simulink model "ASM1_Influentmodel_calibration"  (Simulink 7.6)
settings: Solver=ode45  StartTime=0.0  StopTime=730  RelTol=1e-6
values from neighbouring files (symbols this model uses):
  aHpercent = 75    [ASM1_Influent_init.m]    (also in ASM1_Influent_init_MC_IBU.m; ASM1_Influent_init_MC_T.m; ASM1_Influent_init_MC_TSS.m; ASM1_Influent_init_dry.m)
  CODpart_gperPEperd = 115.08    [ASM1_Influent_init.m]    (also in ASM1_Influent_init_MC_IBU.m; ASM1_Influent_init_MC_T.m = 80; ASM1_Influent_init_MC_TSS.m = RandomMatrix1(a,1); ASM1_Influent_init_dry.m)
  CODpart_HH_max = 20*CODpart_gperPEperd*PE    (= 184128)    [ASM1_Influent_init.m]    (also in ASM1_Influent_init_MC_IBU.m = 36825.6; ASM1_Influent_init_MC_T.m = 25600; ASM1_Influent_init_MC_TSS.m = 20*CODpart_gperPEperd*PE; ASM1_Influent_init_dry.m = 36825.6)
  CODpart_HH_min = 0.1    [ASM1_Influent_init.m]    (also in ASM1_Influent_init_MC_IBU.m; ASM1_Influent_init_MC_T.m; ASM1_Influent_init_MC_TSS.m; ASM1_Influent_init_dry.m)
  CODpart_HH_ns = 35000    [ASM1_Influent_init.m]    (also in ASM1_Influent_init_MC_IBU.m; ASM1_Influent_init_MC_T.m; ASM1_Influent_init_MC_TSS.m; ASM1_Influent_init_dry.m)
  CODpart_HH_nv = factor1*CODpart_gperPEperd*PE    (= 18412.8)    [ASM1_Influent_init.m]    (also in ASM1_Influent_init_MC_IBU.m = 3682.56; ASM1_Influent_init_MC_T.m = 2560; ASM1_Influent_init_MC_TSS.m = factor1*CODpart_gperPEperd*PE; ASM1_Influent_init_dry.m = 3682.56)
  CODpart_HH_st = 1/24    (= 0.0416666666667)    [ASM1_Influent_init.m]    (also in ASM1_Influent_init_MC_IBU.m; ASM1_Influent_init_MC_T.m; ASM1_Influent_init_MC_TSS.m; ASM1_Influent_init_dry.m)
  CODpart_Ind_kgperd = 2301.80    (= 2301.8)    [ASM1_Influent_init.m]    (also in ASM1_Influent_init_MC_IBU.m = 0; ASM1_Influent_init_MC_T.m = 0; ASM1_Influent_init_MC_TSS.m = 0; ASM1_Influent_init_dry.m)
  CODpart_Ind_max = 20*CODpart_Ind_kgperd    (= 46036)    [ASM1_Influent_init.m]    (also in ASM1_Influent_init_MC_IBU.m = 20; ASM1_Influent_init_MC_T.m = 20; ASM1_Influent_init_MC_TSS.m = 20; ASM1_Influent_init_dry.m)
  CODpart_Ind_min = 0.1    [ASM1_Influent_init.m]    (also in ASM1_Influent_init_MC_IBU.m; ASM1_Influent_init_MC_T.m; ASM1_Influent_init_MC_TSS.m; ASM1_Influent_init_dry.m)
  CODpart_Ind_ns = 21000    [ASM1_Influent_init.m]    (also in ASM1_Influent_init_MC_IBU.m; ASM1_Influent_init_MC_T.m; ASM1_Influent_init_MC_TSS.m; ASM1_Influent_init_dry.m)
  CODpart_Ind_nv = factor2*CODpart_Ind_kgperd    (= 4603.6)    [ASM1_Influent_init.m]    (also in ASM1_Influent_init_MC_IBU.m = 0; ASM1_Influent_init_MC_T.m = 0; ASM1_Influent_init_MC_TSS.m = 0; ASM1_Influent_init_dry.m)
  CODpart_Ind_st = 1/24    (= 0.0416666666667)    [ASM1_Influent_init.m]    (also in ASM1_Influent_init_MC_IBU.m; ASM1_Influent_init_MC_T.m; ASM1_Influent_init_MC_TSS.m; ASM1_Influent_init_dry.m)
  CODsol_gperPEperd = 19.31    [ASM1_Influent_init.m]    (also in ASM1_Influent_init_MC_IBU.m; ASM1_Influent_init_MC_T.m; ASM1_Influent_init_MC_TSS.m; ASM1_Influent_init_dry.m)
  CODsol_HH_max = 20*CODsol_gperPEperd*PE    (= 30896)    [ASM1_Influent_init.m]    (also in ASM1_Influent_init_MC_IBU.m = 6179.2; ASM1_Influent_init_MC_T.m = 6179.2; ASM1_Influent_init_MC_TSS.m = 6179.2; ASM1_Influent_init_dry.m = 6179.2)
  CODsol_HH_min = 0.1    [ASM1_Influent_init.m]    (also in ASM1_Influent_init_MC_IBU.m; ASM1_Influent_init_MC_T.m; ASM1_Influent_init_MC_TSS.m; ASM1_Influent_init_dry.m)
  CODsol_HH_ns = 25000    [ASM1_Influent_init.m]    (also in ASM1_Influent_init_MC_IBU.m; ASM1_Influent_init_MC_T.m; ASM1_Influent_init_MC_TSS.m; ASM1_Influent_init_dry.m)
  CODsol_HH_nv = factor1*2*CODsol_gperPEperd*PE    (= 6179.2)    [ASM1_Influent_init.m]    (also in ASM1_Influent_init_MC_IBU.m = 1235.84; ASM1_Influent_init_MC_T.m = 1235.84; ASM1_Influent_init_MC_TSS.m = 1235.84; ASM1_Influent_init_dry.m = 1235.84)
  CODsol_HH_st = 1/24    (= 0.0416666666667)    [ASM1_Influent_init.m]    (also in ASM1_Influent_init_MC_IBU.m; ASM1_Influent_init_MC_T.m; ASM1_Influent_init_MC_TSS.m; ASM1_Influent_init_dry.m)
  CODsol_Ind_kgperd = 386.24    [ASM1_Influent_init.m]    (also in ASM1_Influent_init_MC_IBU.m = 0; ASM1_Influent_init_MC_T.m = 0; ASM1_Influent_init_MC_TSS.m = 0; ASM1_Influent_init_dry.m)
  CODsol_Ind_max = 20*CODsol_Ind_kgperd    (= 7724.8)    [ASM1_Influent_init.m]    (also in ASM1_Influent_init_MC_IBU.m = 20; ASM1_Influent_init_MC_T.m = 20; ASM1_Influent_init_MC_TSS.m = 20; ASM1_Influent_init_dry.m)
  CODsol_Ind_min = 0.1    [ASM1_Influent_init.m]    (also in ASM1_Influent_init_MC_IBU.m; ASM1_Influent_init_MC_T.m; ASM1_Influent_init_MC_TSS.m; ASM1_Influent_init_dry.m)
  CODsol_Ind_ns = 11000    [ASM1_Influent_init.m]    (also in ASM1_Influent_init_MC_IBU.m; ASM1_Influent_init_MC_T.m; ASM1_Influent_init_MC_TSS.m; ASM1_Influent_init_dry.m)
  CODsol_Ind_nv = factor2*CODsol_Ind_kgperd    (= 772.48)    [ASM1_Influent_init.m]    (also in ASM1_Influent_init_MC_IBU.m = 0; ASM1_Influent_init_MC_T.m = 0; ASM1_Influent_init_MC_TSS.m = 0; ASM1_Influent_init_dry.m)
  CODsol_Ind_st = 1/24    (= 0.0416666666667)    [ASM1_Influent_init.m]    (also in ASM1_Influent_init_MC_IBU.m; ASM1_Influent_init_MC_T.m; ASM1_Influent_init_MC_TSS.m; ASM1_Influent_init_dry.m)
  FFfraction = 0.25    [ASM1_Influent_init.m]    (also in ASM1_Influent_init_MC_IBU.m; ASM1_Influent_init_MC_T.m = 0.4; ASM1_Influent_init_MC_TSS.m = RandomMatrix1(a,2); ASM1_Influent_init_dry.m)
  HHnoiseswitch = 1    [ASM1_Influent_init.m]    (also in ASM1_Influent_init_MC_IBU.m; ASM1_Influent_init_MC_T.m; ASM1_Influent_init_MC_TSS.m; ASM1_Influent_init_dry.m)
  HHpolnoiseswitch = 1    [ASM1_Influent_init.m]    (also in ASM1_Influent_init_MC_IBU.m; ASM1_Influent_init_MC_T.m; ASM1_Influent_init_MC_TSS.m; ASM1_Influent_init_dry.m)
  HHpopswitch = 100    [ASM1_Influent_init.m]    (also in ASM1_Influent_init_MC_IBU.m; ASM1_Influent_init_MC_T.m; ASM1_Influent_init_MC_TSS.m; ASM1_Influent_init_dry.m)
  Indnoiseswitch = 1    [ASM1_Influent_init.m]    (also in ASM1_Influent_init_MC_IBU.m; ASM1_Influent_init_MC_T.m; ASM1_Influent_init_MC_TSS.m; ASM1_Influent_init_dry.m)
  Indpolnoiseswitch = 1    [ASM1_Influent_init.m]    (also in ASM1_Influent_init_MC_IBU.m; ASM1_Influent_init_MC_T.m; ASM1_Influent_init_MC_TSS.m; ASM1_Influent_init_dry.m)
  Indpopswitch = 100    [ASM1_Influent_init.m]    (also in ASM1_Influent_init_MC_IBU.m; ASM1_Influent_init_MC_T.m = 0; ASM1_Influent_init_MC_TSS.m = 0; ASM1_Influent_init_dry.m)
  InfAmp = 1200    [ASM1_Influent_init.m]    (also in ASM1_Influent_init_MC_IBU.m; ASM1_Influent_init_MC_T.m; ASM1_Influent_init_MC_TSS.m; ASM1_Influent_init_dry.m)
  InfBias = 7100    [ASM1_Influent_init.m]    (also in ASM1_Influent_init_MC_IBU.m; ASM1_Influent_init_MC_T.m; ASM1_Influent_init_MC_TSS.m; ASM1_Influent_init_dry.m)
  Infcst = 7100    [ASM1_Influent_init.m]    (also in ASM1_Influent_init_MC_IBU.m; ASM1_Influent_init_MC_T.m; ASM1_Influent_init_MC_TSS.m; ASM1_Influent_init_dry.m)
  InfFreq = 2*pi/364    (= 0.0172614980966)    [ASM1_Influent_init.m]    (also in ASM1_Influent_init_MC_IBU.m; ASM1_Influent_init_MC_T.m; ASM1_Influent_init_MC_TSS.m; ASM1_Influent_init_dry.m)
  InfPhase = -pi*15/24    (= -1.96349540849)    [ASM1_Influent_init.m]    (also in ASM1_Influent_init_MC_IBU.m; ASM1_Influent_init_MC_T.m; ASM1_Influent_init_MC_TSS.m; ASM1_Influent_init_dry.m)
  PE = 80    [ASM1_Influent_init.m]    (also in ASM1_Influent_init_MC_IBU.m = 16; ASM1_Influent_init_MC_T.m = 16; ASM1_Influent_init_MC_TSS.m = 16; ASM1_Influent_init_dry.m = 16)
  polnoiseswitch = 1    [ASM1_Influent_init.m]    (also in ASM1_Influent_init_MC_IBU.m; ASM1_Influent_init_MC_T.m; ASM1_Influent_init_MC_TSS.m; ASM1_Influent_init_dry.m)
  Q_HH_ns = 3857    [ASM1_Influent_init.m]    (also in ASM1_Influent_init_MC_IBU.m; ASM1_Influent_init_MC_T.m; ASM1_Influent_init_MC_TSS.m; ASM1_Influent_init_dry.m)
  Q_HH_nv = 4000    [ASM1_Influent_init.m]    (also in ASM1_Influent_init_MC_IBU.m; ASM1_Influent_init_MC_T.m; ASM1_Influent_init_MC_TSS.m; ASM1_Influent_init_dry.m)
  Q_HH_st = 1/24    (= 0.0416666666667)    [ASM1_Influent_init.m]    (also in ASM1_Influent_init_MC_IBU.m; ASM1_Influent_init_MC_T.m; ASM1_Influent_init_MC_TSS.m; ASM1_Influent_init_dry.m)
  Q_Ind_ns = 2000    [ASM1_Influent_init.m]    (also in ASM1_Influent_init_MC_IBU.m; ASM1_Influent_init_MC_T.m; ASM1_Influent_init_MC_TSS.m; ASM1_Influent_init_dry.m)
  Q_Ind_nv = 15000    [ASM1_Influent_init.m]    (also in ASM1_Influent_init_MC_IBU.m; ASM1_Influent_init_MC_T.m; ASM1_Influent_init_MC_TSS.m; ASM1_Influent_init_dry.m)
  Q_Ind_st = 1/24    (= 0.0416666666667)    [ASM1_Influent_init.m]    (also in ASM1_Influent_init_MC_IBU.m; ASM1_Influent_init_MC_T.m; ASM1_Influent_init_MC_TSS.m; ASM1_Influent_init_dry.m)
  Q_SCI_ns = 1000    [ASM1_Influent_init.m]    (also in ASM1_Influent_init_MC_IBU.m; ASM1_Influent_init_MC_T.m; ASM1_Influent_init_MC_TSS.m; ASM1_Influent_init_dry.m)
  Q_SCI_nv = 0.1*InfBias    (= 710)    [ASM1_Influent_init.m]    (also in ASM1_Influent_init_MC_IBU.m; ASM1_Influent_init_MC_T.m; ASM1_Influent_init_MC_TSS.m; ASM1_Influent_init_dry.m)
  Q_SCI_st = 1    [ASM1_Influent_init.m]    (also in ASM1_Influent_init_MC_IBU.m; ASM1_Influent_init_MC_T.m; ASM1_Influent_init_MC_TSS.m; ASM1_Influent_init_dry.m)
  QHHsatmax = QperPE*50    (= 7500)    [ASM1_Influent_init.m]    (also in ASM1_Influent_init_MC_IBU.m; ASM1_Influent_init_MC_T.m; ASM1_Influent_init_MC_TSS.m; ASM1_Influent_init_dry.m)
  QHHsatmin = 0.001    [ASM1_Influent_init.m]    (also in ASM1_Influent_init_MC_IBU.m; ASM1_Influent_init_MC_T.m; ASM1_Influent_init_MC_TSS.m; ASM1_Influent_init_dry.m)
  QInd_weekday = 2500    [ASM1_Influent_init.m]    (also in ASM1_Influent_init_MC_IBU.m; ASM1_Influent_init_MC_T.m; ASM1_Influent_init_MC_TSS.m; ASM1_Influent_init_dry.m)
  QIndsatmax = QInd_weekday*10    (= 25000)    [ASM1_Influent_init.m]    (also in ASM1_Influent_init_MC_IBU.m; ASM1_Influent_init_MC_T.m; ASM1_Influent_init_MC_TSS.m; ASM1_Influent_init_dry.m)
  QIndsatmin = 0.001    [ASM1_Influent_init.m]    (also in ASM1_Influent_init_MC_IBU.m; ASM1_Influent_init_MC_T.m; ASM1_Influent_init_MC_TSS.m; ASM1_Influent_init_dry.m)
  Qpermm = 1500    [ASM1_Influent_init.m]    (also in ASM1_Influent_init_MC_IBU.m; ASM1_Influent_init_MC_T.m; ASM1_Influent_init_MC_TSS.m; ASM1_Influent_init_dry.m)
  QperPE = 150    [ASM1_Influent_init.m]    (also in ASM1_Influent_init_MC_IBU.m; ASM1_Influent_init_MC_T.m; ASM1_Influent_init_MC_TSS.m; ASM1_Influent_init_dry.m)
  QSCIsatmax = 2*(InfBias+InfAmp)    (= 16600)    [ASM1_Influent_init.m]    (also in ASM1_Influent_init_MC_IBU.m; ASM1_Influent_init_MC_T.m; ASM1_Influent_init_MC_TSS.m; ASM1_Influent_init_dry.m)
  QSCIsatmin = 0.0    (= 0)    [ASM1_Influent_init.m]    (also in ASM1_Influent_init_MC_IBU.m; ASM1_Influent_init_MC_T.m; ASM1_Influent_init_MC_TSS.m; ASM1_Influent_init_dry.m)
  rainpopswitch = 100    [ASM1_Influent_init.m]    (also in ASM1_Influent_init_MC_IBU.m = 0; ASM1_Influent_init_MC_T.m = 0; ASM1_Influent_init_MC_TSS.m = 0; ASM1_Influent_init_dry.m = 0)
  SCInoiseswitch = 0    [ASM1_Influent_init.m]    (also in ASM1_Influent_init_MC_IBU.m; ASM1_Influent_init_MC_T.m; ASM1_Influent_init_MC_TSS.m; ASM1_Influent_init_dry.m)
  SCIpopswitch = 100    [ASM1_Influent_init.m]    (also in ASM1_Influent_init_MC_IBU.m; ASM1_Influent_init_MC_T.m; ASM1_Influent_init_MC_TSS.m; ASM1_Influent_init_dry.m)
  SI_max = 100*Si_in    (= 3000)    [ASM1_Influent_init.m]    (also in ASM1_Influent_init_MC_IBU.m; ASM1_Influent_init_MC_T.m; ASM1_Influent_init_MC_TSS.m; ASM1_Influent_init_dry.m)
  SI_min = 0.1    [ASM1_Influent_init.m]    (also in ASM1_Influent_init_MC_IBU.m; ASM1_Influent_init_MC_T.m; ASM1_Influent_init_MC_TSS.m; ASM1_Influent_init_dry.m)
  SI_ns = 13122    [ASM1_Influent_init.m]    (also in ASM1_Influent_init_MC_IBU.m; ASM1_Influent_init_MC_T.m; ASM1_Influent_init_MC_TSS.m; ASM1_Influent_init_dry.m)
  SI_nv = factor3*(Si_in)    (= 60)    [ASM1_Influent_init.m]    (also in ASM1_Influent_init_MC_IBU.m; ASM1_Influent_init_MC_T.m; ASM1_Influent_init_MC_TSS.m; ASM1_Influent_init_dry.m)
  SI_st = 1/24    (= 0.0416666666667)    [ASM1_Influent_init.m]    (also in ASM1_Influent_init_MC_IBU.m; ASM1_Influent_init_MC_T.m; ASM1_Influent_init_MC_TSS.m; ASM1_Influent_init_dry.m)
  SND_max = 100*Snd_in    (= 695)    [ASM1_Influent_init.m]    (also in ASM1_Influent_init_MC_IBU.m; ASM1_Influent_init_MC_T.m; ASM1_Influent_init_MC_TSS.m; ASM1_Influent_init_dry.m)
  SND_min = 0.1    [ASM1_Influent_init.m]    (also in ASM1_Influent_init_MC_IBU.m; ASM1_Influent_init_MC_T.m; ASM1_Influent_init_MC_TSS.m; ASM1_Influent_init_dry.m)
  SND_ns = 73122    [ASM1_Influent_init.m]    (also in ASM1_Influent_init_MC_IBU.m; ASM1_Influent_init_MC_T.m; ASM1_Influent_init_MC_TSS.m; ASM1_Influent_init_dry.m)
  SND_nv = factor3*(Snd_in)    (= 13.9)    [ASM1_Influent_init.m]    (also in ASM1_Influent_init_MC_IBU.m; ASM1_Influent_init_MC_T.m; ASM1_Influent_init_MC_TSS.m; ASM1_Influent_init_dry.m)
  SND_st = 1/24    (= 0.0416666666667)    [ASM1_Influent_init.m]    (also in ASM1_Influent_init_MC_IBU.m; ASM1_Influent_init_MC_T.m; ASM1_Influent_init_MC_TSS.m; ASM1_Influent_init_dry.m)
  SNH_gperPEperd = 6.89*0.85    (= 5.8565)    [ASM1_Influent_init.m]    (also in ASM1_Influent_init_MC_IBU.m = 6.36; ASM1_Influent_init_MC_T.m = 6.37; ASM1_Influent_init_MC_TSS.m = 6.37; ASM1_Influent_init_dry.m = 6.36)
  SNH_HH_max = 20*SNH_gperPEperd*PE    (= 9370.4)    [ASM1_Influent_init.m]    (also in ASM1_Influent_init_MC_IBU.m = 101760; ASM1_Influent_init_MC_T.m = 101920; ASM1_Influent_init_MC_TSS.m = 101920; ASM1_Influent_init_dry.m = 2035.2)
  SNH_HH_min = 0.1    [ASM1_Influent_init.m]    (also in ASM1_Influent_init_MC_IBU.m; ASM1_Influent_init_MC_T.m; ASM1_Influent_init_MC_TSS.m; ASM1_Influent_init_dry.m)
  SNH_HH_ns = 45000    [ASM1_Influent_init.m]    (also in ASM1_Influent_init_MC_IBU.m; ASM1_Influent_init_MC_T.m; ASM1_Influent_init_MC_TSS.m; ASM1_Influent_init_dry.m)
  SNH_HH_nv = factor1*2*SNH_gperPEperd*PE    (= 1874.08)    [ASM1_Influent_init.m]    (also in ASM1_Influent_init_MC_IBU.m = 407.04; ASM1_Influent_init_MC_T.m = 407.68; ASM1_Influent_init_MC_TSS.m = 407.68; ASM1_Influent_init_dry.m = 407.04)
  SNH_HH_st = 1/24    (= 0.0416666666667)    [ASM1_Influent_init.m]    (also in ASM1_Influent_init_MC_IBU.m; ASM1_Influent_init_MC_T.m; ASM1_Influent_init_MC_TSS.m; ASM1_Influent_init_dry.m)
  SNH_Ind_kgperd = 61.25*0.85    (= 52.0625)    [ASM1_Influent_init.m]    (also in ASM1_Influent_init_MC_IBU.m = 0; ASM1_Influent_init_MC_T.m = 0; ASM1_Influent_init_MC_TSS.m = 0; ASM1_Influent_init_dry.m)
  SNH_Ind_max = 20*SNH_Ind_kgperd    (= 1041.25)    [ASM1_Influent_init.m]    (also in ASM1_Influent_init_MC_IBU.m = 20; ASM1_Influent_init_MC_T.m = 20; ASM1_Influent_init_MC_TSS.m = 20; ASM1_Influent_init_dry.m)
  SNH_Ind_min = 0.1    [ASM1_Influent_init.m]    (also in ASM1_Influent_init_MC_IBU.m; ASM1_Influent_init_MC_T.m; ASM1_Influent_init_MC_TSS.m; ASM1_Influent_init_dry.m)
  SNH_Ind_ns = 31000    [ASM1_Influent_init.m]    (also in ASM1_Influent_init_MC_IBU.m; ASM1_Influent_init_MC_T.m; ASM1_Influent_init_MC_TSS.m; ASM1_Influent_init_dry.m)
  SNH_Ind_nv = factor2*SNH_Ind_kgperd    (= 104.125)    [ASM1_Influent_init.m]    (also in ASM1_Influent_init_MC_IBU.m = 0; ASM1_Influent_init_MC_T.m = 0; ASM1_Influent_init_MC_TSS.m = 0; ASM1_Influent_init_dry.m)
  SNH_Ind_st = 1/24    (= 0.0416666666667)    [ASM1_Influent_init.m]    (also in ASM1_Influent_init_MC_IBU.m; ASM1_Influent_init_MC_T.m; ASM1_Influent_init_MC_TSS.m; ASM1_Influent_init_dry.m)
  SNH_max = 100*Snh_in    (= 3156)    [ASM1_Influent_init.m]    (also in ASM1_Influent_init_MC_IBU.m; ASM1_Influent_init_MC_T.m; ASM1_Influent_init_MC_TSS.m; ASM1_Influent_init_dry.m)
  SNH_min = 0.1    [ASM1_Influent_init.m]    (also in ASM1_Influent_init_MC_IBU.m; ASM1_Influent_init_MC_T.m; ASM1_Influent_init_MC_TSS.m; ASM1_Influent_init_dry.m)
  SNH_ns = 63122    [ASM1_Influent_init.m]    (also in ASM1_Influent_init_MC_IBU.m; ASM1_Influent_init_MC_T.m; ASM1_Influent_init_MC_TSS.m; ASM1_Influent_init_dry.m)
  SNH_nv = factor3*(Snh_in)    (= 63.12)    [ASM1_Influent_init.m]    (also in ASM1_Influent_init_MC_IBU.m; ASM1_Influent_init_MC_T.m; ASM1_Influent_init_MC_TSS.m; ASM1_Influent_init_dry.m)
  SNH_st = 1/24    (= 0.0416666666667)    [ASM1_Influent_init.m]    (also in ASM1_Influent_init_MC_IBU.m; ASM1_Influent_init_MC_T.m; ASM1_Influent_init_MC_TSS.m; ASM1_Influent_init_dry.m)
  SS_max = 100*Ss_in    (= 6950)    [ASM1_Influent_init.m]    (also in ASM1_Influent_init_MC_IBU.m; ASM1_Influent_init_MC_T.m; ASM1_Influent_init_MC_TSS.m; ASM1_Influent_init_dry.m)
  SS_min = 0.1    [ASM1_Influent_init.m]    (also in ASM1_Influent_init_MC_IBU.m; ASM1_Influent_init_MC_T.m; ASM1_Influent_init_MC_TSS.m; ASM1_Influent_init_dry.m)
  SS_ns = 23122    [ASM1_Influent_init.m]    (also in ASM1_Influent_init_MC_IBU.m; ASM1_Influent_init_MC_T.m; ASM1_Influent_init_MC_TSS.m; ASM1_Influent_init_dry.m)
  SS_nv = factor3*(Ss_in)    (= 139)    [ASM1_Influent_init.m]    (also in ASM1_Influent_init_MC_IBU.m; ASM1_Influent_init_MC_T.m; ASM1_Influent_init_MC_TSS.m; ASM1_Influent_init_dry.m)
  SS_st = 1/24    (= 0.0416666666667)    [ASM1_Influent_init.m]    (also in ASM1_Influent_init_MC_IBU.m; ASM1_Influent_init_MC_T.m; ASM1_Influent_init_MC_TSS.m; ASM1_Influent_init_dry.m)
  subareas = 4    [ASM1_Influent_init.m]    (also in ASM1_Influent_init_MC_IBU.m = round(RandomMatrix1(a,4)); ASM1_Influent_init_MC_T.m; ASM1_Influent_init_MC_TSS.m; ASM1_Influent_init_dry.m)
  TAmp = 5    [ASM1_Influent_init.m]    (also in ASM1_Influent_init_MC_IBU.m; ASM1_Influent_init_MC_T.m = RandomMatrix1(a,1); ASM1_Influent_init_MC_TSS.m; ASM1_Influent_init_dry.m)
  TBias = 15    [ASM1_Influent_init.m]    (also in ASM1_Influent_init_MC_IBU.m; ASM1_Influent_init_MC_T.m = RandomMatrix1(a,2); ASM1_Influent_init_MC_TSS.m = 18; ASM1_Influent_init_dry.m)
  TdAmp = 0.5    [ASM1_Influent_init.m]    (also in ASM1_Influent_init_MC_IBU.m; ASM1_Influent_init_MC_T.m = RandomMatrix1(a,3); ASM1_Influent_init_MC_TSS.m = 0.6; ASM1_Influent_init_dry.m)
  TdBias = 0    [ASM1_Influent_init.m]    (also in ASM1_Influent_init_MC_IBU.m; ASM1_Influent_init_MC_T.m; ASM1_Influent_init_MC_TSS.m; ASM1_Influent_init_dry.m)
  TdFreq = 2*pi    (= 6.28318530718)    [ASM1_Influent_init.m]    (also in ASM1_Influent_init_MC_IBU.m; ASM1_Influent_init_MC_T.m; ASM1_Influent_init_MC_TSS.m; ASM1_Influent_init_dry.m)
  TdPhase = pi*0.8    (= 2.51327412287)    [ASM1_Influent_init.m]    (also in ASM1_Influent_init_MC_IBU.m; ASM1_Influent_init_MC_T.m; ASM1_Influent_init_MC_TSS.m; ASM1_Influent_init_dry.m)
  TFreq = 2*pi/364    (= 0.0172614980966)    [ASM1_Influent_init.m]    (also in ASM1_Influent_init_MC_IBU.m; ASM1_Influent_init_MC_T.m; ASM1_Influent_init_MC_TSS.m; ASM1_Influent_init_dry.m)
  TKN_gperPEperd = 14.24*0.85    (= 12.104)    [ASM1_Influent_init.m]    (also in ASM1_Influent_init_MC_IBU.m = 14.24; ASM1_Influent_init_MC_T.m = 14.24; ASM1_Influent_init_MC_TSS.m = 14.24; ASM1_Influent_init_dry.m = 14.24)
  TKN_HH_max = 20*TKN_gperPEperd*PE    (= 19366.4)    [ASM1_Influent_init.m]    (also in ASM1_Influent_init_MC_IBU.m = 4556.8; ASM1_Influent_init_MC_T.m = 4556.8; ASM1_Influent_init_MC_TSS.m = 4556.8; ASM1_Influent_init_dry.m = 4556.8)
  TKN_HH_min = 0.1    [ASM1_Influent_init.m]    (also in ASM1_Influent_init_MC_IBU.m; ASM1_Influent_init_MC_T.m; ASM1_Influent_init_MC_TSS.m; ASM1_Influent_init_dry.m)
  TKN_HH_ns = 55000    [ASM1_Influent_init.m]    (also in ASM1_Influent_init_MC_IBU.m; ASM1_Influent_init_MC_T.m; ASM1_Influent_init_MC_TSS.m; ASM1_Influent_init_dry.m)
  TKN_HH_nv = factor1*1.5*TKN_gperPEperd*PE    (= 2904.96)    [ASM1_Influent_init.m]    (also in ASM1_Influent_init_MC_IBU.m = 683.52; ASM1_Influent_init_MC_T.m = 683.52; ASM1_Influent_init_MC_TSS.m = 683.52; ASM1_Influent_init_dry.m = 683.52)
  TKN_HH_st = 1/24    (= 0.0416666666667)    [ASM1_Influent_init.m]    (also in ASM1_Influent_init_MC_IBU.m; ASM1_Influent_init_MC_T.m; ASM1_Influent_init_MC_TSS.m; ASM1_Influent_init_dry.m)
  TKN_Ind_kgperd = 128.62*0.85    (= 109.327)    [ASM1_Influent_init.m]    (also in ASM1_Influent_init_MC_IBU.m = 0; ASM1_Influent_init_MC_T.m = 0; ASM1_Influent_init_MC_TSS.m = 0; ASM1_Influent_init_dry.m)
  TKN_Ind_max = 20*TKN_Ind_kgperd    (= 2186.54)    [ASM1_Influent_init.m]    (also in ASM1_Influent_init_MC_IBU.m = 20; ASM1_Influent_init_MC_T.m = 20; ASM1_Influent_init_MC_TSS.m = 20; ASM1_Influent_init_dry.m)
  TKN_Ind_min = 0.1    [ASM1_Influent_init.m]    (also in ASM1_Influent_init_MC_IBU.m; ASM1_Influent_init_MC_T.m; ASM1_Influent_init_MC_TSS.m; ASM1_Influent_init_dry.m)
  TKN_Ind_ns = 41000    [ASM1_Influent_init.m]    (also in ASM1_Influent_init_MC_IBU.m; ASM1_Influent_init_MC_T.m; ASM1_Influent_init_MC_TSS.m; ASM1_Influent_init_dry.m)
  TKN_Ind_nv = factor2*TKN_Ind_kgperd    (= 218.654)    [ASM1_Influent_init.m]    (also in ASM1_Influent_init_MC_IBU.m = 0; ASM1_Influent_init_MC_T.m = 0; ASM1_Influent_init_MC_TSS.m = 0; ASM1_Influent_init_dry.m)
  TKN_Ind_st = 1/24    (= 0.0416666666667)    [ASM1_Influent_init.m]    (also in ASM1_Influent_init_MC_IBU.m; ASM1_Influent_init_MC_T.m; ASM1_Influent_init_MC_TSS.m; ASM1_Influent_init_dry.m)
  TPhase = pi*8.5/24    (= 1.11264739815)    [ASM1_Influent_init.m]    (also in ASM1_Influent_init_MC_IBU.m; ASM1_Influent_init_MC_T.m = 3.14159265359; ASM1_Influent_init_MC_TSS.m; ASM1_Influent_init_dry.m)
  X_BA2TSS = 0.75    [ASM1_Influent_init.m]    (also in ASM1_Influent_init_MC_IBU.m; ASM1_Influent_init_MC_T.m; ASM1_Influent_init_MC_TSS.m; ASM1_Influent_init_dry.m)
  X_BH2TSS = 0.75    [ASM1_Influent_init.m]    (also in ASM1_Influent_init_MC_IBU.m; ASM1_Influent_init_MC_T.m; ASM1_Influent_init_MC_TSS.m; ASM1_Influent_init_dry.m)
  X_I2TSS = 0.75    [ASM1_Influent_init.m]    (also in ASM1_Influent_init_MC_IBU.m; ASM1_Influent_init_MC_T.m; ASM1_Influent_init_MC_TSS.m; ASM1_Influent_init_dry.m)
  X_P2TSS = 0.75    [ASM1_Influent_init.m]    (also in ASM1_Influent_init_MC_IBU.m; ASM1_Influent_init_MC_T.m; ASM1_Influent_init_MC_TSS.m; ASM1_Influent_init_dry.m)
  X_S2TSS = 0.75    [ASM1_Influent_init.m]    (also in ASM1_Influent_init_MC_IBU.m; ASM1_Influent_init_MC_T.m; ASM1_Influent_init_MC_TSS.m; ASM1_Influent_init_dry.m)
  XBH_max = 200*Xbh_in    (= 5634)    [ASM1_Influent_init.m]    (also in ASM1_Influent_init_MC_IBU.m; ASM1_Influent_init_MC_T.m; ASM1_Influent_init_MC_TSS.m; ASM1_Influent_init_dry.m)
  XBH_min = 0.1    [ASM1_Influent_init.m]    (also in ASM1_Influent_init_MC_IBU.m; ASM1_Influent_init_MC_T.m; ASM1_Influent_init_MC_TSS.m; ASM1_Influent_init_dry.m)
  ... (+18 more)
undefined symbols (not defined in the file or in its folder): filter, Qpersnow, samplingtime
libraries: simulink x1
(part 2 of 2)

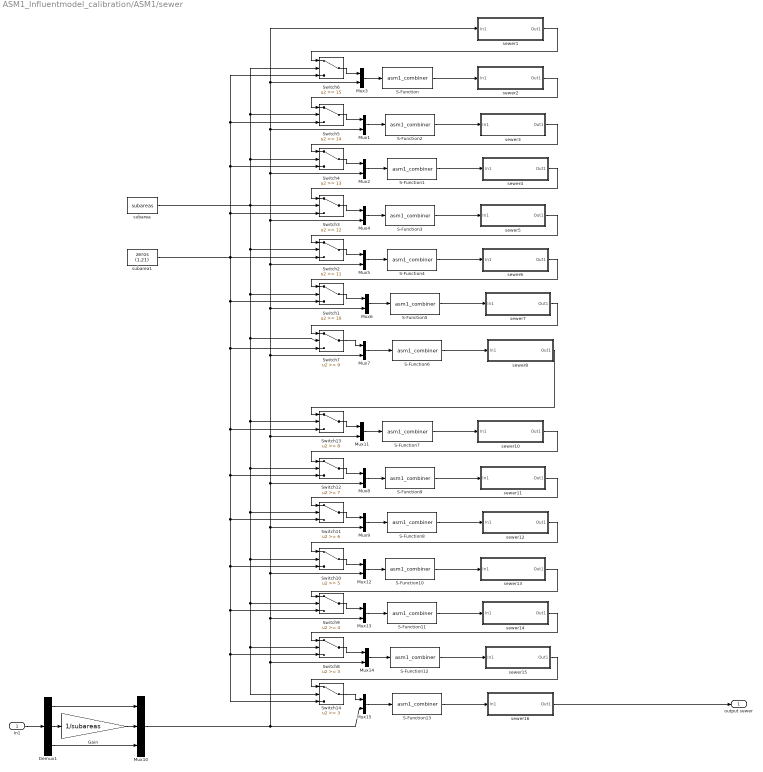
== system ASM1_Influentmodel_calibration/ASM1/sewer ==
  In1 : Inport
  Demux1 : Demux  Outputs=[14 1 6]
  Gain : Gain  Gain=1/subareas
  Mux{1..9,11..15} (14 alike) : Mux  Inputs=2
  Mux10 : Mux  Inputs=3
  S-Function{,1..13} (14 alike) : S-Function  FunctionName=asm1_combiner  EnableBusSupport=off
  Switch1 : Switch  Threshold=10  SaturateOnIntegerOverflow=on
  Switch10 : Switch  Threshold=5  SaturateOnIntegerOverflow=on
  Switch11 : Switch  Threshold=6  SaturateOnIntegerOverflow=on
  Switch12 : Switch  Threshold=7  SaturateOnIntegerOverflow=on
  Switch13 : Switch  Threshold=8  SaturateOnIntegerOverflow=on
  Switch14 : Switch  Threshold=3  SaturateOnIntegerOverflow=on
  Switch2 : Switch  Threshold=11  SaturateOnIntegerOverflow=on
  Switch3 : Switch  Threshold=12  SaturateOnIntegerOverflow=on
  Switch4 : Switch  Threshold=13  SaturateOnIntegerOverflow=on
  Switch5 : Switch  Threshold=14  SaturateOnIntegerOverflow=on
  Switch6 : Switch  Threshold=15  SaturateOnIntegerOverflow=on
  Switch7 : Switch  Threshold=9  SaturateOnIntegerOverflow=on
  Switch8 : Switch  Threshold=3  SaturateOnIntegerOverflow=on
  Switch9 : Switch  Threshold=4  SaturateOnIntegerOverflow=on
  sewer1 : Subsystem
  sewer10 : Subsystem
  sewer11 : Subsystem
  sewer12 : Subsystem
  sewer13 : Subsystem
  sewer14 : Subsystem
  sewer15 : Subsystem
  sewer16 : Subsystem
  sewer2 : Subsystem
  sewer3 : Subsystem
  sewer4 : Subsystem
  sewer5 : Subsystem
  sewer6 : Subsystem
  sewer7 : Subsystem
  sewer8 : Subsystem
  subarea : Constant  Value=subareas
  subarea1 : Constant  Value=zeros (1,21)
  output sewer : Outport
  wires:
  In1/1 -> Demux1/1
  Demux1/2 -> Gain/1
  Demux1/1 -> Mux10/1
  Demux1/3 -> Mux10/3
  Gain/1 -> Mux10/2
  S-Function/1 -> sewer2/1(In1)
  sewer2/1(Out1) -> Switch5/1
  S-Function2/1 -> sewer3/1(In1)
  sewer3/1(Out1) -> Switch4/1
  S-Function1/1 -> sewer4/1(In1)
  sewer4/1(Out1) -> Switch3/1
  S-Function3/1 -> sewer5/1(In1)
  sewer5/1(Out1) -> Switch2/1
  sewer1/1(Out1) -> Switch6/1
  S-Function4/1 -> sewer6/1(In1)
  sewer6/1(Out1) -> Switch1/1
  S-Function5/1 -> sewer7/1(In1)
  sewer7/1(Out1) -> Switch7/1
  S-Function6/1 -> sewer8/1(In1)
  Switch6/1 -> Mux3/1
  Mux3/1 -> S-Function/1
  Switch5/1 -> Mux1/1
  Switch4/1 -> Mux2/1
  Switch3/1 -> Mux4/1
  Switch1/1 -> Mux6/1
  Switch2/1 -> Mux5/1
  Switch7/1 -> Mux7/1
  Mux1/1 -> S-Function2/1
  Mux2/1 -> S-Function1/1
  Mux4/1 -> S-Function3/1
  Mux5/1 -> S-Function4/1
  Mux6/1 -> S-Function5/1
  Mux7/1 -> S-Function6/1
  subarea/1 -> Switch3/2, Switch6/2, Switch5/2, Switch4/2, Switch2/2, Switch1/2, Switch7/2, Switch13/2, Switch12/2, Switch11/2, Switch10/2, Switch9/2, Switch8/2, Switch14/2
  subarea1/1 -> Switch2/3, Switch6/3, Switch5/3, Switch4/3, Switch3/3, Switch1/3, Switch7/3, Switch13/3, Switch12/3, Switch11/3, Switch10/3, Switch9/3, Switch8/3, Switch14/3
  S-Function7/1 -> sewer10/1(In1)
  sewer10/1(Out1) -> Switch12/1
  S-Function9/1 -> sewer11/1(In1)
  sewer11/1(Out1) -> Switch11/1
  S-Function8/1 -> sewer12/1(In1)
  sewer12/1(Out1) -> Switch10/1
  S-Function10/1 -> sewer13/1(In1)
  sewer13/1(Out1) -> Switch9/1
  S-Function11/1 -> sewer14/1(In1)
  sewer14/1(Out1) -> Switch8/1
  S-Function12/1 -> sewer15/1(In1)
  sewer15/1(Out1) -> Switch14/1
  S-Function13/1 -> sewer16/1(In1)
  Switch13/1 -> Mux11/1
  Mux11/1 -> S-Function7/1
  Switch12/1 -> Mux8/1
  Switch11/1 -> Mux9/1
  Switch10/1 -> Mux12/1
  Switch8/1 -> Mux14/1
  Switch9/1 -> Mux13/1
  Switch14/1 -> Mux15/1
  Mux8/1 -> S-Function9/1
  Mux9/1 -> S-Function8/1
  Mux12/1 -> S-Function10/1
  Mux13/1 -> S-Function11/1
  Mux14/1 -> S-Function12/1
  Mux15/1 -> S-Function13/1
  sewer16/1(Out1) -> output sewer/1
  sewer8/1(Out1) -> Switch13/1
  Mux10/1 -> Mux15/2, Mux14/2, Mux13/2, Mux12/2, Mux9/2, Mux8/2, Mux7/2, Mux6/2, Mux5/2, Mux4/2, sewer1/1(In1), Mux3/2, Mux1/2, Mux2/2, Mux11/2

== system ASM1_Influentmodel_calibration/Rain generation flow rate  model block/T filter ==
  In1 : Inport
  In2 : Inport  Port=2
  Add : Sum
  Constant3 : Constant  Value=1-1/(filter*(1440/samplingtime))
  Constant4 : Constant  Value=(1-(1-1/(filter*(1440/samplingtime))))
  Product1 : Product  RndMeth=Zero
  Product2 : Product  RndMeth=Zero
  Unit Delay : UnitDelay  SampleTime=(1/96)
  Out1 : Outport
  wires:
  In2/1 -> Product2/1
  Constant3/1 -> Product1/2
  Unit Delay/1 -> Product1/1
  Constant4/1 -> Product2/2
  Product1/1 -> Add/1
  Product2/1 -> Add/2
  Add/1 -> Out1/1
  In1/1 -> Unit Delay/1

== system ASM1_Influentmodel_calibration/ASM1/Noise application/Add noise SI ==
  In1 : Inport
  Random Number : RandomNumber  Variance=SI_nv*polnoiseswitch  Seed=SI_ns  SampleTime=SI_st
  Saturation : Saturate  UpperLimit=SI_max  LowerLimit=SI_min
  Sum : Sum  Inputs=|++  SaturateOnIntegerOverflow=on
  Out1 : Outport
  wires:
  Sum/1 -> Saturation/1
  Random Number/1 -> Sum/2
  Saturation/1 -> Out1/1
  In1/1 -> Sum/1

== system ASM1_Influentmodel_calibration/ASM1/Noise application/Add noise SND ==
  In1 : Inport
  Random Number : RandomNumber  Variance=SND_nv*polnoiseswitch  Seed=SND_ns  SampleTime=SND_st
  Saturation : Saturate  UpperLimit=SND_max  LowerLimit=SND_min
  Sum : Sum  Inputs=|++  SaturateOnIntegerOverflow=on
  Out1 : Outport
  wires:
  Sum/1 -> Saturation/1
  Random Number/1 -> Sum/2
  Saturation/1 -> Out1/1
  In1/1 -> Sum/1

== system ASM1_Influentmodel_calibration/ASM1/Noise application/Add noise SNH ==
  In1 : Inport
  Random Number : RandomNumber  Variance=SNH_nv*polnoiseswitch  Seed=SNH_ns  SampleTime=SNH_st
  Saturation : Saturate  UpperLimit=SNH_max  LowerLimit=SNH_min
  Sum : Sum  Inputs=|++  SaturateOnIntegerOverflow=on
  Out1 : Outport
  wires:
  Sum/1 -> Saturation/1
  Random Number/1 -> Sum/2
  Saturation/1 -> Out1/1
  In1/1 -> Sum/1

== system ASM1_Influentmodel_calibration/ASM1/Noise application/Add noise SS ==
  In1 : Inport
  Random Number : RandomNumber  Variance=SS_nv*polnoiseswitch  Seed=SS_ns  SampleTime=SS_st
  Saturation : Saturate  UpperLimit=SS_max  LowerLimit=SS_min
  Sum : Sum  Inputs=|++  SaturateOnIntegerOverflow=on
  Out1 : Outport
  wires:
  Sum/1 -> Saturation/1
  Random Number/1 -> Sum/2
  Saturation/1 -> Out1/1
  In1/1 -> Sum/1

== system ASM1_Influentmodel_calibration/ASM1/Noise application/Add noise XBH ==
  In1 : Inport
  Random Number : RandomNumber  Variance=XBH_nv*polnoiseswitch  Seed=XBH_ns  SampleTime=XBH_st
  Saturation : Saturate  UpperLimit=XBH_max  LowerLimit=XBH_min
  Sum : Sum  Inputs=|++  SaturateOnIntegerOverflow=on
  Out1 : Outport
  wires:
  Sum/1 -> Saturation/1
  Random Number/1 -> Sum/2
  Saturation/1 -> Out1/1
  In1/1 -> Sum/1

== system ASM1_Influentmodel_calibration/ASM1/Noise application/Add noise XI ==
  In1 : Inport
  Random Number : RandomNumber  Variance=XI_nv*polnoiseswitch  Seed=XI_ns  SampleTime=XI_st
  Saturation : Saturate  UpperLimit=XI_max  LowerLimit=XI_min
  Sum : Sum  Inputs=|++  SaturateOnIntegerOverflow=on
  Out1 : Outport
  wires:
  Sum/1 -> Saturation/1
  Random Number/1 -> Sum/2
  Saturation/1 -> Out1/1
  In1/1 -> Sum/1

== system ASM1_Influentmodel_calibration/ASM1/Noise application/Add noise XND ==
  In1 : Inport
  Random Number : RandomNumber  Variance=XND_nv*polnoiseswitch  Seed=XND_ns  SampleTime=XND_st
  Saturation : Saturate  UpperLimit=XND_max  LowerLimit=XND_min
  Sum : Sum  Inputs=|++  SaturateOnIntegerOverflow=on
  Out1 : Outport
  wires:
  Sum/1 -> Saturation/1
  Random Number/1 -> Sum/2
  Saturation/1 -> Out1/1
  In1/1 -> Sum/1

== system ASM1_Influentmodel_calibration/ASM1/Noise application/Add noise XS ==
  In1 : Inport
  Random Number : RandomNumber  Variance=XS_nv*polnoiseswitch  Seed=XS_ns  SampleTime=XS_st
  Saturation : Saturate  UpperLimit=XS_max  LowerLimit=XS_min
  Sum : Sum  Inputs=|++  SaturateOnIntegerOverflow=on
  Out1 : Outport
  wires:
  Sum/1 -> Saturation/1
  Random Number/1 -> Sum/2
  Saturation/1 -> Out1/1
  In1/1 -> Sum/1

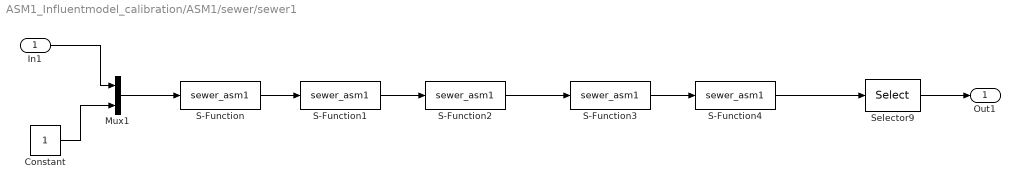
== system ASM1_Influentmodel_calibration/ASM1/sewer/sewer1 ==
  In1 : Inport
  Constant : Constant
  Mux1 : Mux  Inputs=2
  S-Function{,1..4} (5 alike) : S-Function  FunctionName=sewer_asm1  Parameters=ASM1_SEWERINIT, ASM1_PARS, SPAR  EnableBusSupport=off
  Selector9 : Selector  InputPortWidth=22  IndexOptions=Index vector (dialog)  Indices=[1 2 3 4 5 6 7 8 9 10 11 12 13 14 15 16 17 18 19 20 21]  OutputSizes=1
  Out1 : Outport
  wires:
  S-Function/1 -> S-Function1/1
  S-Function1/1 -> S-Function2/1
  Mux1/1 -> S-Function/1
  Constant/1 -> Mux1/2
  In1/1 -> Mux1/1
  Selector9/1 -> Out1/1
  S-Function3/1 -> S-Function4/1
  S-Function2/1 -> S-Function3/1
  S-Function4/1 -> Selector9/1

== system ASM1_Influentmodel_calibration/ASM1/sewer/sewer10 ==
  In1 : Inport
  Constant : Constant
  Mux1 : Mux  Inputs=2
  S-Function{,1..4} (5 alike) : S-Function  FunctionName=sewer_asm1  Parameters=ASM1_SEWERINIT, ASM1_PARS, SPAR  EnableBusSupport=off
  Selector9 : Selector  InputPortWidth=22  IndexOptions=Index vector (dialog)  Indices=[1 2 3 4 5 6 7 8 9 10 11 12 13 14 15 16 17 18 19 20 21]  OutputSizes=1
  Out1 : Outport
  wires:
  S-Function/1 -> S-Function1/1
  S-Function1/1 -> S-Function2/1
  Mux1/1 -> S-Function/1
  Constant/1 -> Mux1/2
  Selector9/1 -> Out1/1
  In1/1 -> Mux1/1
  S-Function3/1 -> S-Function4/1
  S-Function2/1 -> S-Function3/1
  S-Function4/1 -> Selector9/1

== system ASM1_Influentmodel_calibration/ASM1/sewer/sewer11 ==
  In1 : Inport
  Constant : Constant
  Mux1 : Mux  Inputs=2
  S-Function{,1..4} (5 alike) : S-Function  FunctionName=sewer_asm1  Parameters=ASM1_SEWERINIT, ASM1_PARS, SPAR  EnableBusSupport=off
  Selector9 : Selector  InputPortWidth=22  IndexOptions=Index vector (dialog)  Indices=[1 2 3 4 5 6 7 8 9 10 11 12 13 14 15 16 17 18 19 20 21]  OutputSizes=1
  Out1 : Outport
  wires:
  S-Function/1 -> S-Function1/1
  S-Function1/1 -> S-Function2/1
  Mux1/1 -> S-Function/1
  Constant/1 -> Mux1/2
  In1/1 -> Mux1/1
  Selector9/1 -> Out1/1
  S-Function3/1 -> S-Function4/1
  S-Function2/1 -> S-Function3/1
  S-Function4/1 -> Selector9/1

== system ASM1_Influentmodel_calibration/ASM1/sewer/sewer12 ==
  In1 : Inport
  Constant : Constant
  Mux1 : Mux  Inputs=2
  S-Function{,1..4} (5 alike) : S-Function  FunctionName=sewer_asm1  Parameters=ASM1_SEWERINIT, ASM1_PARS, SPAR  EnableBusSupport=off
  Selector9 : Selector  InputPortWidth=22  IndexOptions=Index vector (dialog)  Indices=[1 2 3 4 5 6 7 8 9 10 11 12 13 14 15 16 17 18 19 20 21]  OutputSizes=1
  Out1 : Outport
  wires:
  S-Function/1 -> S-Function1/1
  S-Function1/1 -> S-Function2/1
  Mux1/1 -> S-Function/1
  Constant/1 -> Mux1/2
  In1/1 -> Mux1/1
  Selector9/1 -> Out1/1
  S-Function3/1 -> S-Function4/1
  S-Function2/1 -> S-Function3/1
  S-Function4/1 -> Selector9/1

== system ASM1_Influentmodel_calibration/ASM1/sewer/sewer13 ==
  In1 : Inport
  Constant : Constant
  Mux1 : Mux  Inputs=2
  S-Function{,1..4} (5 alike) : S-Function  FunctionName=sewer_asm1  Parameters=ASM1_SEWERINIT, ASM1_PARS, SPAR  EnableBusSupport=off
  Selector9 : Selector  InputPortWidth=22  IndexOptions=Index vector (dialog)  Indices=[1 2 3 4 5 6 7 8 9 10 11 12 13 14 15 16 17 18 19 20 21]  OutputSizes=1
  Out1 : Outport
  wires:
  S-Function/1 -> S-Function1/1
  S-Function1/1 -> S-Function2/1
  Mux1/1 -> S-Function/1
  Constant/1 -> Mux1/2
  In1/1 -> Mux1/1
  Selector9/1 -> Out1/1
  S-Function3/1 -> S-Function4/1
  S-Function2/1 -> S-Function3/1
  S-Function4/1 -> Selector9/1

== system ASM1_Influentmodel_calibration/ASM1/sewer/sewer14 ==
  In1 : Inport
  Constant : Constant
  Mux1 : Mux  Inputs=2
  S-Function{,1..4} (5 alike) : S-Function  FunctionName=sewer_asm1  Parameters=ASM1_SEWERINIT, ASM1_PARS, SPAR  EnableBusSupport=off
  Selector9 : Selector  InputPortWidth=22  IndexOptions=Index vector (dialog)  Indices=[1 2 3 4 5 6 7 8 9 10 11 12 13 14 15 16 17 18 19 20 21]  OutputSizes=1
  Out1 : Outport
  wires:
  S-Function/1 -> S-Function1/1
  S-Function1/1 -> S-Function2/1
  Mux1/1 -> S-Function/1
  Constant/1 -> Mux1/2
  In1/1 -> Mux1/1
  Selector9/1 -> Out1/1
  S-Function3/1 -> S-Function4/1
  S-Function2/1 -> S-Function3/1
  S-Function4/1 -> Selector9/1

== system ASM1_Influentmodel_calibration/ASM1/sewer/sewer15 ==
  In1 : Inport
  Constant : Constant
  Mux1 : Mux  Inputs=2
  S-Function{,1..4} (5 alike) : S-Function  FunctionName=sewer_asm1  Parameters=ASM1_SEWERINIT, ASM1_PARS, SPAR  EnableBusSupport=off
  Selector9 : Selector  InputPortWidth=22  IndexOptions=Index vector (dialog)  Indices=[1 2 3 4 5 6 7 8 9 10 11 12 13 14 15 16 17 18 19 20 21]  OutputSizes=1
  Out1 : Outport
  wires:
  S-Function/1 -> S-Function1/1
  S-Function1/1 -> S-Function2/1
  Mux1/1 -> S-Function/1
  Constant/1 -> Mux1/2
  In1/1 -> Mux1/1
  Selector9/1 -> Out1/1
  S-Function3/1 -> S-Function4/1
  S-Function2/1 -> S-Function3/1
  S-Function4/1 -> Selector9/1

== system ASM1_Influentmodel_calibration/ASM1/sewer/sewer16 ==
  In1 : Inport
  Constant : Constant
  Mux1 : Mux  Inputs=2
  S-Function{,1..4} (5 alike) : S-Function  FunctionName=sewer_asm1  Parameters=ASM1_SEWERINIT, ASM1_PARS, SPAR  EnableBusSupport=off
  Selector9 : Selector  InputPortWidth=22  IndexOptions=Index vector (dialog)  Indices=[1 2 3 4 5 6 7 8 9 10 11 12 13 14 15 16 17 18 19 20 21]  OutputSizes=1
  Out1 : Outport
  wires:
  S-Function/1 -> S-Function1/1
  S-Function1/1 -> S-Function2/1
  Mux1/1 -> S-Function/1
  Constant/1 -> Mux1/2
  In1/1 -> Mux1/1
  Selector9/1 -> Out1/1
  S-Function3/1 -> S-Function4/1
  S-Function2/1 -> S-Function3/1
  S-Function4/1 -> Selector9/1

== system ASM1_Influentmodel_calibration/ASM1/sewer/sewer2 ==
  In1 : Inport
  Constant : Constant
  Mux1 : Mux  Inputs=2
  S-Function{,1..4} (5 alike) : S-Function  FunctionName=sewer_asm1  Parameters=ASM1_SEWERINIT, ASM1_PARS, SPAR  EnableBusSupport=off
  Selector9 : Selector  InputPortWidth=22  IndexOptions=Index vector (dialog)  Indices=[1 2 3 4 5 6 7 8 9 10 11 12 13 14 15 16 17 18 19 20 21]  OutputSizes=1
  Out1 : Outport
  wires:
  S-Function/1 -> S-Function1/1
  S-Function1/1 -> S-Function2/1
  Mux1/1 -> S-Function/1
  Constant/1 -> Mux1/2
  Selector9/1 -> Out1/1
  In1/1 -> Mux1/1
  S-Function3/1 -> S-Function4/1
  S-Function2/1 -> S-Function3/1
  S-Function4/1 -> Selector9/1

== system ASM1_Influentmodel_calibration/ASM1/sewer/sewer3 ==
  In1 : Inport
  Constant : Constant
  Mux1 : Mux  Inputs=2
  S-Function{,1..4} (5 alike) : S-Function  FunctionName=sewer_asm1  Parameters=ASM1_SEWERINIT, ASM1_PARS, SPAR  EnableBusSupport=off
  Selector9 : Selector  InputPortWidth=22  IndexOptions=Index vector (dialog)  Indices=[1 2 3 4 5 6 7 8 9 10 11 12 13 14 15 16 17 18 19 20 21]  OutputSizes=1
  Out1 : Outport
  wires:
  S-Function/1 -> S-Function1/1
  S-Function1/1 -> S-Function2/1
  Mux1/1 -> S-Function/1
  Constant/1 -> Mux1/2
  In1/1 -> Mux1/1
  Selector9/1 -> Out1/1
  S-Function3/1 -> S-Function4/1
  S-Function2/1 -> S-Function3/1
  S-Function4/1 -> Selector9/1

== system ASM1_Influentmodel_calibration/ASM1/sewer/sewer4 ==
  In1 : Inport
  Constant : Constant
  Mux1 : Mux  Inputs=2
  S-Function{,1..4} (5 alike) : S-Function  FunctionName=sewer_asm1  Parameters=ASM1_SEWERINIT, ASM1_PARS, SPAR  EnableBusSupport=off
  Selector9 : Selector  InputPortWidth=22  IndexOptions=Index vector (dialog)  Indices=[1 2 3 4 5 6 7 8 9 10 11 12 13 14 15 16 17 18 19 20 21]  OutputSizes=1
  Out1 : Outport
  wires:
  S-Function/1 -> S-Function1/1
  S-Function1/1 -> S-Function2/1
  Mux1/1 -> S-Function/1
  Constant/1 -> Mux1/2
  In1/1 -> Mux1/1
  Selector9/1 -> Out1/1
  S-Function3/1 -> S-Function4/1
  S-Function2/1 -> S-Function3/1
  S-Function4/1 -> Selector9/1

== system ASM1_Influentmodel_calibration/ASM1/sewer/sewer5 ==
  In1 : Inport
  Constant : Constant
  Mux1 : Mux  Inputs=2
  S-Function{,1..4} (5 alike) : S-Function  FunctionName=sewer_asm1  Parameters=ASM1_SEWERINIT, ASM1_PARS, SPAR  EnableBusSupport=off
  Selector9 : Selector  InputPortWidth=22  IndexOptions=Index vector (dialog)  Indices=[1 2 3 4 5 6 7 8 9 10 11 12 13 14 15 16 17 18 19 20 21]  OutputSizes=1
  Out1 : Outport
  wires:
  S-Function/1 -> S-Function1/1
  S-Function1/1 -> S-Function2/1
  Mux1/1 -> S-Function/1
  Constant/1 -> Mux1/2
  In1/1 -> Mux1/1
  Selector9/1 -> Out1/1
  S-Function3/1 -> S-Function4/1
  S-Function2/1 -> S-Function3/1
  S-Function4/1 -> Selector9/1

== system ASM1_Influentmodel_calibration/ASM1/sewer/sewer6 ==
  In1 : Inport
  Constant : Constant
  Mux1 : Mux  Inputs=2
  S-Function{,1..4} (5 alike) : S-Function  FunctionName=sewer_asm1  Parameters=ASM1_SEWERINIT, ASM1_PARS, SPAR  EnableBusSupport=off
  Selector9 : Selector  InputPortWidth=22  IndexOptions=Index vector (dialog)  Indices=[1 2 3 4 5 6 7 8 9 10 11 12 13 14 15 16 17 18 19 20 21]  OutputSizes=1
  Out1 : Outport
  wires:
  S-Function/1 -> S-Function1/1
  S-Function1/1 -> S-Function2/1
  Mux1/1 -> S-Function/1
  Constant/1 -> Mux1/2
  In1/1 -> Mux1/1
  Selector9/1 -> Out1/1
  S-Function3/1 -> S-Function4/1
  S-Function2/1 -> S-Function3/1
  S-Function4/1 -> Selector9/1

== system ASM1_Influentmodel_calibration/ASM1/sewer/sewer7 ==
  In1 : Inport
  Constant : Constant
  Mux1 : Mux  Inputs=2
  S-Function{,1..4} (5 alike) : S-Function  FunctionName=sewer_asm1  Parameters=ASM1_SEWERINIT, ASM1_PARS, SPAR  EnableBusSupport=off
  Selector9 : Selector  InputPortWidth=22  IndexOptions=Index vector (dialog)  Indices=[1 2 3 4 5 6 7 8 9 10 11 12 13 14 15 16 17 18 19 20 21]  OutputSizes=1
  Out1 : Outport
  wires:
  S-Function/1 -> S-Function1/1
  S-Function1/1 -> S-Function2/1
  Mux1/1 -> S-Function/1
  Constant/1 -> Mux1/2
  In1/1 -> Mux1/1
  Selector9/1 -> Out1/1
  S-Function3/1 -> S-Function4/1
  S-Function2/1 -> S-Function3/1
  S-Function4/1 -> Selector9/1

== system ASM1_Influentmodel_calibration/ASM1/sewer/sewer8 ==
  In1 : Inport
  Constant : Constant
  Mux1 : Mux  Inputs=2
  S-Function{,1..4} (5 alike) : S-Function  FunctionName=sewer_asm1  Parameters=ASM1_SEWERINIT, ASM1_PARS, SPAR  EnableBusSupport=off
  Selector9 : Selector  InputPortWidth=22  IndexOptions=Index vector (dialog)  Indices=[1 2 3 4 5 6 7 8 9 10 11 12 13 14 15 16 17 18 19 20 21]  OutputSizes=1
  Out1 : Outport
  wires:
  S-Function/1 -> S-Function1/1
  S-Function1/1 -> S-Function2/1
  Mux1/1 -> S-Function/1
  Constant/1 -> Mux1/2
  In1/1 -> Mux1/1
  Selector9/1 -> Out1/1
  S-Function3/1 -> S-Function4/1
  S-Function2/1 -> S-Function3/1
  S-Function4/1 -> Selector9/1
